simulink library "MT3515"  (R2024a)
settings: Solver=VariableStepAuto  StartTime=0.0  StopTime=10.0  RelTol=1e-3
undefined symbols (not defined in the file): geo, prop
settings Model: Creator=igmso  LastModifiedBy=igmso

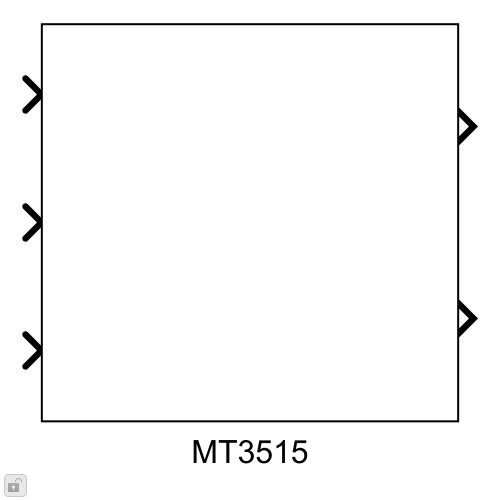
[thumbnail: Simulink's stored preview of the top-level diagram]
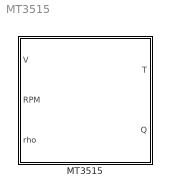
== system MT3515 ==
  MT3515 : Subsystem

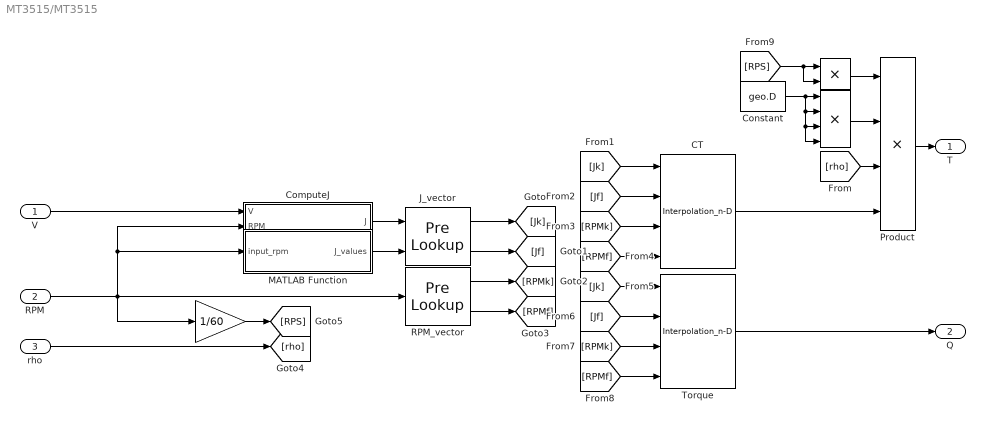
== system MT3515/MT3515 ==
  V : Inport
  RPM : Inport  Port=2
  rho : Inport  Port=3
  " " : Gain  Gain=1/60
  "  " : Product  Inputs=4
  "   " : Product
  CT : Interpolation_n-D  Table=reshape(prop.data(:,2,:),29,[])  ExtrapMethod=Clip
  ComputeJ : Subsystem
  Constant : Constant  Value=geo.D  SampleTime=-1
  J_vector : PreLookup  BreakpointsDataSource=Input port  BreakpointsData=tilt_rpm  IndexSearchMethod=Linear search
      settings: InputPortMap=u0,p1
  MATLAB Function : MATLAB Function  TreatAsAtomicUnit=on
  Product : Product  Inputs=4
  RPM_vector : PreLookup  BreakpointsData=prop.rpm  IndexSearchMethod=Evenly spaced points
  Torque : Interpolation_n-D  Table=reshape(prop.data(:,3,:),29,[])  ExtrapMethod=Clip
  T : Outport
  Q : Outport  Port=2
  wires:
  RPM_vector/1 -> [RPMk]
  [RPS] -> "   "/2, "   "/1
  Product/1 -> T/1
  RPM/1 -> ComputeJ/2(RPM), MATLAB Function/1(input_rpm), " "/1, RPM_vector/1
  [RPMk] -> Torque/3
  J_vector/1 -> [Jk]
  Constant/1 -> "  "/4, "  "/3, "  "/2, "  "/1
  "   "/1 -> Product/1
  J_vector/2 -> [Jf]
  [Jk] -> CT/1
  rho/1 -> [rho]
  [rho] -> Product/3
  MATLAB Function/1(J_values) -> J_vector/2
  RPM_vector/2 -> [RPMf]
  V/1 -> ComputeJ/1(V)
  "  "/1 -> Product/2
  [Jf] -> Torque/2
  ComputeJ/1(J) -> J_vector/1
  " "/1 -> [RPS]
  CT/1 -> Product/4
  [RPMk] -> CT/3
  [Jf] -> CT/2
  [RPMf] -> CT/4
  [Jk] -> Torque/1
  [RPMf] -> Torque/4
  Torque/1 -> Q/1

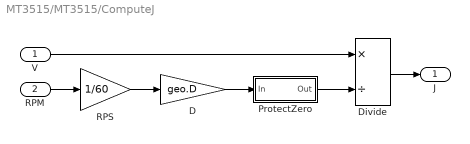
== system MT3515/MT3515/ComputeJ ==
  V : Inport
  RPM : Inport  Port=2
  D : Gain  Gain=geo.D
  Divide : Product  Inputs=*/
  ProtectZero : Subsystem
  RPS : Gain  Gain=1/60
  J : Outport
  wires:
  RPM/1 -> RPS/1
  D/1 -> ProtectZero/1(In)
  RPS/1 -> D/1
  Divide/1 -> J/1
  V/1 -> Divide/1
  ProtectZero/1(Out) -> Divide/2

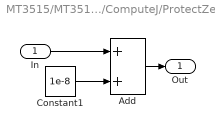
== system MT3515/MT3515/ComputeJ/ProtectZero ==
  In : Inport
  Add : Sum
  Constant1 : Constant  Value=1e-8  SampleTime=-1
  Out : Outport
  wires:
  Constant1/1 -> Add/2
  Add/1 -> Out/1
  In/1 -> Add/1

== matlab function MT3515/MATLAB Function ==
  data: input_rpm input; J_values output
function J_values = get_J_by_rpm(input_rpm)

rpm_values = [1000	3000	5000	7000	9000	11000	13000	15000	17000	19000];

J = [0	0	0	0	0	0	0	0	0	0
0.0169	0.0171	0.0169	0.0173	0.0170	0.0170	0.0171	0.0170	0.0174	0.0172
0.0337	0.0342	0.0339	0.0347	0.0339	0.0339	0.0343	0.0339	0.0347	0.0343
0.0506	0.0514	0.0508	0.0520	0.0509	0.0509	0.0514	0.0509	0.0521	0.0515
0.0674	0.0685	0.0677	0.0694	0.0678	0.0678	0.0685	0.0679	0.0695	0.0687
0.0843	0.0856	0.0847	0.0867	0.0848	0.0848	0.0857	0.0849	0.0868	0.0859
0.1011	0.1027	0.1016	0.1041	0.1017	0.1018	0.1028	0.1018	0.1042	0.103
0.118	0.1198	0.1185	0.1214	0.1187	0.1187	0.1199	0.1188	0.1216	0.1202
0.1349	0.137	0.1354	0.1387	0.1356	0.1357	0.1371	0.1358	0.1389	0.1374
0.1517	0.1541	0.1524	0.1561	0.1526	0.1527	0.1542	0.1528	0.1563	0.1545
0.1686	0.1712	0.1693	0.1734	0.1695	0.1696	0.1714	0.1697	0.1736	0.1717
0.1854	0.1883	0.1862	0.1908	0.1865	0.1866	0.1885	0.1867	0.191	0.1889
0.2023	0.2054	0.2032	0.2081	0.2034	0.2035	0.2056	0.2037	0.2084	0.2061
0.2191	0.2226	0.2201	0.2255	0.2204	0.2205	0.2228	0.2206	0.2257	0.2232
0.236	0.2397	0.237	0.2428	0.2373	0.2375	0.2399	0.2376	0.2431	0.2404
0.2528	0.2568	0.254	0.2601	0.2543	0.2544	0.257	0.2546	0.2605	0.2576
0.2697	0.2739	0.2709	0.2775	0.2712	0.2714	0.2742	0.2716	0.2778	0.2747
0.2866	0.291	0.2878	0.2948	0.2882	0.2884	0.2913	0.2885	0.2952	0.2919
0.3034	0.3081	0.3048	0.3122	0.3051	0.3053	0.3084	0.3055	0.3126	0.3091
0.3203	0.3253	0.3217	0.3295	0.3221	0.3223	0.3256	0.3225	0.3299	0.3263
0.3371	0.3424	0.3386	0.3469	0.339	0.3392	0.3427	0.3395	0.3473	0.3434
0.354	0.3595	0.3555	0.3642	0.356	0.3562	0.3598	0.3564	0.3647	0.3606
0.3708	0.3766	0.3725	0.3815	0.3729	0.3732	0.377	0.3734	0.382	0.3778
0.3877	0.3937	0.3894	0.3989	0.3899	0.3901	0.3941	0.3904	0.3994	0.395
0.4046	0.4109	0.4063	0.4162	0.4068	0.4071	0.4112	0.4073	0.4167	0.4121
0.4214	0.428	0.4233	0.4336	0.4238	0.4241	0.4284	0.4243	0.4341	0.4293
0.4383	0.4451	0.4402	0.4509	0.4407	0.441	0.4455	0.4413	0.4515	0.4465
0.4551	0.4622	0.4571	0.4683	0.4577	0.458	0.4627	0.4583	0.4688	0.4636
0.472	0.4793	0.4741	0.4856	0.4746	0.4749	0.4798	0.4752	0.4862	0.4808];

% Encontra o índice do RPM mais próximo
[~, closest_index] = min(abs(rpm_values - input_rpm));
    
% Seleciona a coluna correspondente da matriz J
J_values = J(:, closest_index);
end
